simulink model "idc2ff_digital_09"  (Simulink 8.7)
settings: Solver=ode45  StartTime=0.0  StopTime=10.0  RelTol=1e-3
undefined symbols (not defined in the file or in its folder): M, OSR, tclk
libraries: dspsigops x5
settings Model: Creator=chench  LastModifiedBy=Derek
settings DataIOCC: SignalLoggingSaveFormat=ModelDataLogs
settings OptimizationCC: ExpressionDepthLimit=2147483647  InitFltsAndDblsToZero=on
settings DebuggingCC: SaveWithParameterizedLinksMsg=none  SignalResolutionControl=TryResolveAllWithWarning  SolverPrmCheckMsg=warning  MultiTaskDSMMsg=warning  MultiTaskCondExecSysMsg=none  FcnCallInpInsideContextMsg=UseLocalSettings  StateNameClashWarn=warning  StrictBusMsg=None
settings GRTTargetCC: TargetFcnLib=ansi_tfl_tmw.mat  CombineOutputUpdateFcns=off  GRTInterface=on

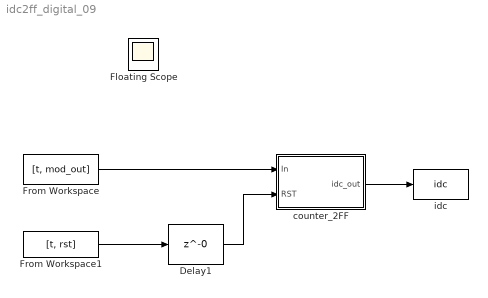
== system idc2ff_digital_09 ==
  Delay1 : Delay  DelayLength=0  InitialCondition=0  InputProcessing=Inherited
  From Workspace : FromWorkspace  VariableName=[t, mod_out]  SampleTime=tclk  Interpolate=off  OutputAfterFinalValue=Holding final value
  From Workspace1 : FromWorkspace  VariableName=[t, rst]  SampleTime=tclk  Interpolate=off  OutputAfterFinalValue=Holding final value
  counter_2FF : Subsystem
  idc : ToWorkspace  VariableName=idc  SampleTime=-1
  Floating Scope : Scope
  wires:
  From Workspace/1 -> counter_2FF/1(In)
  counter_2FF/1(idc_out) -> idc/1
  From Workspace1/1 -> Delay1/1
  Delay1/1 -> counter_2FF/2(RST)

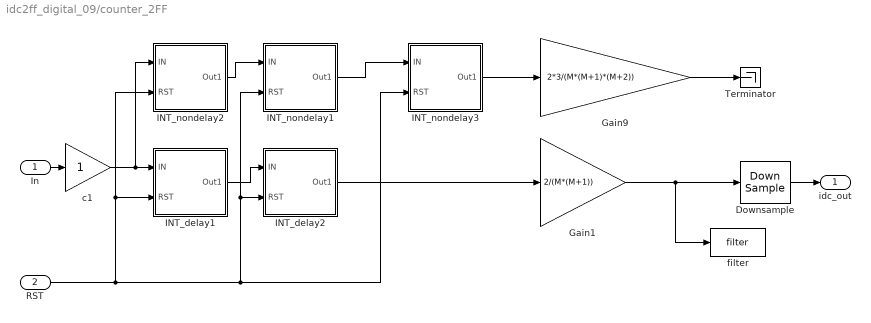
== system idc2ff_digital_09/counter_2FF ==
  In : Inport
  RST : Inport  Port=2
  Downsample : DownSample  N=OSR  phase=OSR-1  InputProcessing=Inherited (this choice will be removed - see release notes)
  Gain1 : Gain  Gain=2/(M*(M+1))
  Gain9 : Gain  Gain=2*3/(M*(M+1)*(M+2))
  INT_delay1 : Subsystem
  INT_delay2 : Subsystem
  INT_nondelay1 : Subsystem
  INT_nondelay2 : Subsystem
  INT_nondelay3 : Subsystem
  Terminator : Terminator
  c1 : Gain  SaturateOnIntegerOverflow=on  OutDataTypeStr=Inherit: Same as input  ParamDataTypeStr=Inherit: Same as input
  filter : ToWorkspace  VariableName=filter  SampleTime=-1
  idc_out : Outport
  wires:
  RST/1 -> INT_delay1/2(RST), INT_nondelay2/2(RST), INT_delay2/2(RST), INT_nondelay1/2(RST), INT_nondelay3/2(RST)
  Downsample/1 -> idc_out/1
  c1/1 -> INT_delay1/1(IN), INT_nondelay2/1(IN)
  In/1 -> c1/1
  INT_delay1/1(Out1) -> INT_delay2/1(IN)
  INT_nondelay2/1(Out1) -> INT_nondelay1/1(IN)
  INT_nondelay1/1(Out1) -> INT_nondelay3/1(IN)
  INT_nondelay3/1(Out1) -> Gain9/1
  Gain1/1 -> filter/1, Downsample/1
  INT_delay2/1(Out1) -> Gain1/1
  Gain9/1 -> Terminator/1

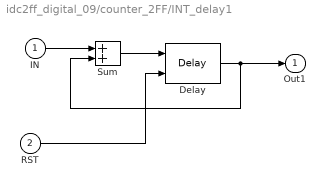
== system idc2ff_digital_09/counter_2FF/INT_delay1 ==
  IN : Inport
  RST : Inport  Port=2
  Delay : dspsigops/Delay  InputProcessing=Inherited (this choice will be removed - see release notes)  dly_unit=Samples  delay=1  ic_detail=off  dif_ic_for_ch=off  dif_ic_for_dly=off  ic=0  reset_popup=Non-zero sample
  Sum : Sum  SaturateOnIntegerOverflow=on  InputSameDT=on  OutDataTypeStr=Inherit: Same as first input
  Out1 : Outport
  wires:
  IN/1 -> Sum/1
  RST/1 -> Delay/2
  Delay/1 -> Sum/2, Out1/1
  Sum/1 -> Delay/1

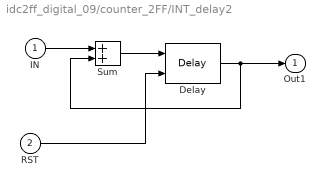
== system idc2ff_digital_09/counter_2FF/INT_delay2 ==
  IN : Inport
  RST : Inport  Port=2
  Delay : dspsigops/Delay  InputProcessing=Inherited (this choice will be removed - see release notes)  dly_unit=Samples  delay=1  ic_detail=off  dif_ic_for_ch=off  dif_ic_for_dly=off  ic=0  reset_popup=Non-zero sample
  Sum : Sum  SaturateOnIntegerOverflow=on  InputSameDT=on  OutDataTypeStr=Inherit: Same as first input
  Out1 : Outport
  wires:
  IN/1 -> Sum/1
  RST/1 -> Delay/2
  Delay/1 -> Sum/2, Out1/1
  Sum/1 -> Delay/1

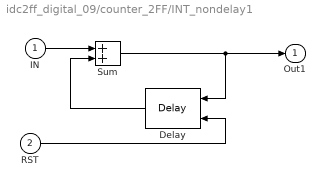
== system idc2ff_digital_09/counter_2FF/INT_nondelay1 ==
  IN : Inport
  RST : Inport  Port=2
  Delay : dspsigops/Delay  InputProcessing=Inherited (this choice will be removed - see release notes)  dly_unit=Samples  delay=1  ic_detail=off  dif_ic_for_ch=off  dif_ic_for_dly=off  ic=0  reset_popup=Non-zero sample
  Sum : Sum  SaturateOnIntegerOverflow=on  InputSameDT=on  OutDataTypeStr=Inherit: Same as first input
  Out1 : Outport
  wires:
  IN/1 -> Sum/1
  Sum/1 -> Out1/1, Delay/1
  RST/1 -> Delay/2
  Delay/1 -> Sum/2

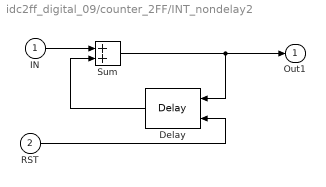
== system idc2ff_digital_09/counter_2FF/INT_nondelay2 ==
  IN : Inport
  RST : Inport  Port=2
  Delay : dspsigops/Delay  InputProcessing=Inherited (this choice will be removed - see release notes)  dly_unit=Samples  delay=1  ic_detail=off  dif_ic_for_ch=off  dif_ic_for_dly=off  ic=0  reset_popup=Non-zero sample
  Sum : Sum  SaturateOnIntegerOverflow=on  InputSameDT=on  OutDataTypeStr=Inherit: Same as first input
  Out1 : Outport
  wires:
  IN/1 -> Sum/1
  Sum/1 -> Out1/1, Delay/1
  RST/1 -> Delay/2
  Delay/1 -> Sum/2

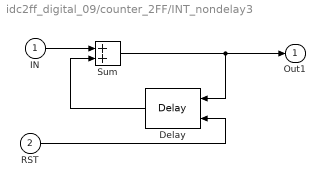
== system idc2ff_digital_09/counter_2FF/INT_nondelay3 ==
  IN : Inport
  RST : Inport  Port=2
  Delay : dspsigops/Delay  InputProcessing=Inherited (this choice will be removed - see release notes)  dly_unit=Samples  delay=1  ic_detail=off  dif_ic_for_ch=off  dif_ic_for_dly=off  ic=0  reset_popup=Non-zero sample
  Sum : Sum  SaturateOnIntegerOverflow=on  InputSameDT=on  OutDataTypeStr=Inherit: Same as first input
  Out1 : Outport
  wires:
  IN/1 -> Sum/1
  Sum/1 -> Out1/1, Delay/1
  RST/1 -> Delay/2
  Delay/1 -> Sum/2
